simulink model "PID_flam_Matlab"  (R2017a)
settings: Solver=VariableStepAuto  StartTime=0.0  StopTime=10.0  RelTol=1e-3
libraries: simulink x1
settings Model: Creator=robotica  LastModifiedBy=robotica

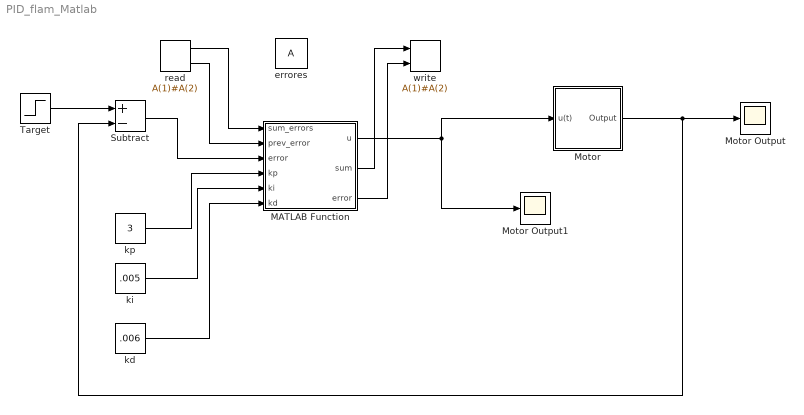
== system PID_flam_Matlab ==
  MATLAB Function : MATLAB Function  TreatAsAtomicUnit=on
  Motor : Subsystem
  Motor Output : Scope
  Motor Output1 : Scope
  Subtract : Sum  Inputs=+-
  Target : Step  SampleTime=1
  errores : DataStoreMemory  ReadBeforeWriteMsg=warning  WriteAfterWriteMsg=warning  WriteAfterReadMsg=warning  InitialValue=[0,0]  ShowAdditionalParam=off  Dimensions=2
  kd : Constant  Value=.006
  ki : Constant  Value=.005
  "kp " : Constant  Value=3
  read : DataStoreRead  DataStoreElements=A(1)#A(2)
  write : DataStoreWrite  DataStoreElements=A(1)#A(2)
  wires:
  Target/1 -> Subtract/1
  Motor/1(Output) -> Subtract/2, Motor Output/1
  MATLAB Function/1(u) -> Motor Output1/1, Motor/1(u(t))
  MATLAB Function/2(sum) -> write/1
  "kp "/1 -> MATLAB Function/4(kp)
  ki/1 -> MATLAB Function/5(ki)
  kd/1 -> MATLAB Function/6(kd)
  read/1 -> MATLAB Function/1(sum_errors)
  read/2 -> MATLAB Function/2(prev_error)
  Subtract/1 -> MATLAB Function/3("error ")
  MATLAB Function/3(error) -> write/2

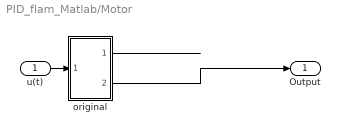
== system PID_flam_Matlab/Motor ==
  u(t) : Inport
  original : Subsystem
  Output : Outport
  wires:
  u(t)/1 -> original/1(signal)
  original/1(noisy) -> ?
  original/2(clean) -> Output/1

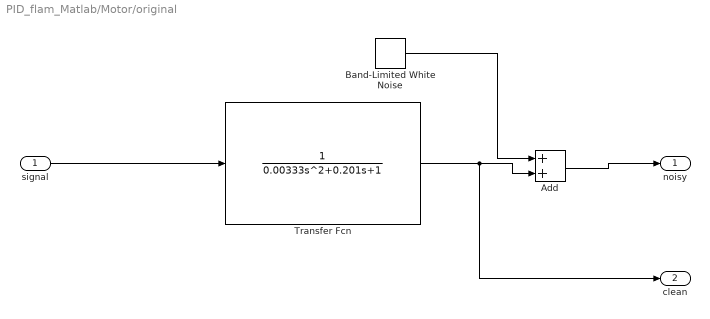
== system PID_flam_Matlab/Motor/original ==
  signal : Inport
  Add : Sum
  Band-Limited White Noise : simulink/Sources/Band-Limited White Noise  Cov=[0.0000001]  Ts=0.001  seed=[23341]
  Transfer Fcn : TransferFcn  Denominator=[0.00333 0.201 1]
  noisy : Outport
  clean : Outport  Port=2
  wires:
  Transfer Fcn/1 -> clean/1, Add/2
  Band-Limited White Noise/1 -> Add/1
  Add/1 -> noisy/1
  signal/1 -> Transfer Fcn/1

== matlab function PID_flam_Matlab/MATLAB Function ==
  data: sum_errors input; prev_error input; error input; u output; kp input; ki input; kd input; sum output; error output
function [u,sum, error]= fcn(sum_errors, prev_error, error,kp, ki, kd)
    p = kp*error;
    
    sum = error + sum_errors;
    i = ki*sum;
    
    dif = error - prev_error;
    d = kd*dif; 
    
    u = p + i +d;
